simulink model "test"  (R2015a)
settings: Solver=ode3  StartTime=0.0  StopTime=inf  FixedStep=0.01  RelTol=1e-3
undefined symbols (not defined in the file or in its folder): Serial_Port, Standard_Devices
libraries: AAxpcseriallibold x2, xpcseriallib x2, simulink x1, xpcobsoletelib x1, sldrtlib x1
settings Model: SimulationMode=external  Creator=mcshardd  LastModifiedBy=mcshardd
settings SolverCC: EnableConcurrentExecution=on
settings OptimizationCC: BlockReduction=off  OptimizeBlockIOStorage=off  BufferReuse=off  GlobalBufferReuse=off  ExpressionFolding=off  LocalBlockOutputs=off
settings HardwareCC: ProdIntDivRoundTo=Zero  ProdEndianess=LittleEndian  ProdLongLongMode=on  ProdHWDeviceType=Generic->32-bit x86 compatible
settings RTWCC: SystemTargetFile=slrt.tlc  TemplateMakefile=slrt_default_tmf  Description=Simulink Real-Time  RTWCompilerOptimization=on
settings SimulinkRealTimeCC: GeneratePreprocessorConditionals=Disable all

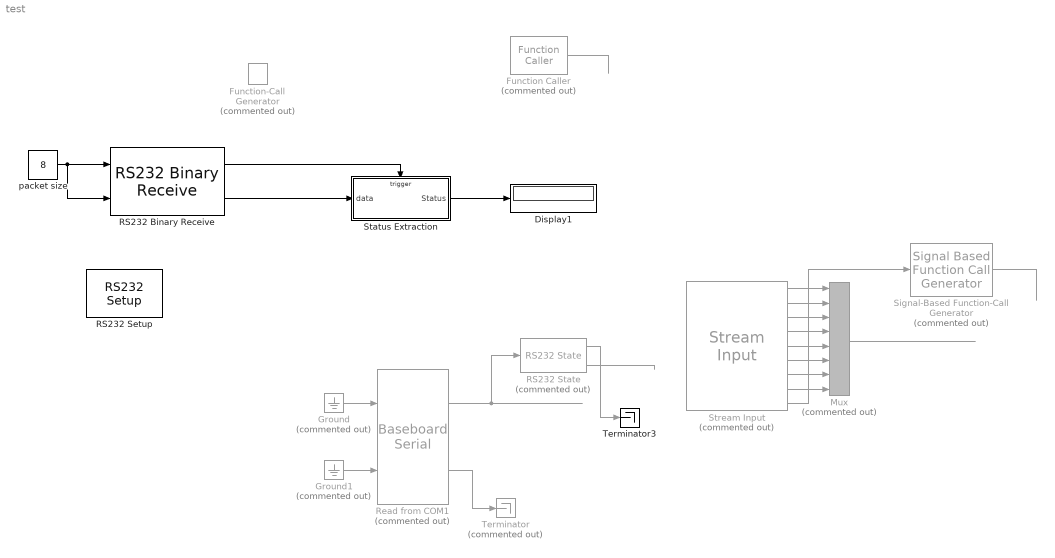
== system test ==
  Display1 : Display
  Function Caller : FunctionCaller  Commented=on  FunctionPrototype=y = f(u)  InputArgumentSpecifications=boolean(1)  OutputArgumentSpecifications=boolean(1)
  Function-Call Generator : simulink/Ports & Subsystems/Function-Call Generator  Commented=on  sample_time=-1  numberOfIterations=1
  Ground : Ground  Commented=on
  Ground1 : Ground  Commented=on
  Mux : Mux  Commented=on  Inputs=8
  RS232 Binary Receive : AAxpcseriallibold/Obsolete/Binary Mode/RS232 Binary Receive  port=COM3  width=8  samptime=-1
  "RS232 Setup " : AAxpcseriallibold/Obsolete/RS232 Setup   port=COM1  baud=19200  dbits=8  sbits=1  parity=None  prot=None  sbuf=2048  rbuf=2048  initstruct=[]  termstruct=[]
  RS232 State : xpcseriallib/RS232 State  Commented=on  overrun=off  parity=off  frame=off  breakint=on
  Read from COM1 : xpcseriallib/Mainboard/Baseboard Serial  Commented=on  group=Receive Setup  port=1  irqnum=4  saddr1=0x3e8  saddr2=0x3e8  config=Custom  baud1=115200  parity1=None  ndata1=8  nstop1=1  fifomode1=16 deep  rlevel1=half full  automode1=off  xmtfifosize1=2048  xmtdatatype1=8 bit uint null terminated  rcvfifosize1=2048  rcvmaxread1=2048  rcvminread1=1  rcvusedelim1=on  rcvdelim1=13  rcvdatatype1=8 bit int null terminated  rcvsampletime1=-1  baud2=115200  parity2=None  ndata2=8  nstop2=1  fifomode2=16 deep  rlevel2=half full  automode2=off  xmtfifosize2=1024  xmtdatatype2=8 bit uint null terminated  rcvfifosize2=1024  rcvmaxread2=1024  rcvminread2=1  rcvusedelim2=on  rcvdelim2=13  rcvdatatype2=count+16 bit uint  rcvsampletime2=.01
      link override FIFO read 1: enable=off
  Signal-Based Function-Call Generator : SignalBasedFunctionCallGenerator  Commented=on  GenerateFunctionCallUpon=Trigger from port tr
      settings: InputPortMap=u1
  Status Extraction : Subsystem  TreatAsAtomicUnit=on
  Stream Input : sldrtlib/Stream Input  Commented=on  SampleTime=0.1  MaxMissedTicks=10  ShowMissedTicks=off  YieldWhenWaiting=off  DrvName=Standard_Devices/Serial_Port  DrvAddress=1  DrvOptions=[115200 8 0 0 0 0 0 0]  DataTypes={'double' 'double' 'double' 'double' 'double' 'double' 'double' 'double'}  FormatString="'%f %f %f %f %f %f  %f %f'"  Terminator={'\r', '\n'}  ShowReady=on  ShowError=off
      settings: AttributesFormatString=Standard Devices\nSerial Port [1h]
  Terminator : Terminator  Commented=on
  Terminator3 : Terminator
  packet size : Constant  Value=8
  wires:
  Status Extraction/1(Status) -> Display1/1
  Stream Input/1 -> Mux/1
  Stream Input/2 -> Mux/2
  Stream Input/3 -> Mux/3
  Stream Input/4 -> Mux/4
  Stream Input/5 -> Mux/5
  Stream Input/6 -> Mux/6
  Stream Input/7 -> Mux/7
  Stream Input/8 -> Mux/8
  Stream Input/9 -> Signal-Based Function-Call Generator/1
  Mux/1 -> ?
  Signal-Based Function-Call Generator/1 -> ?
  Read from COM1/1 -> RS232 State/1
  Ground/1 -> Read from COM1/1
  Read from COM1/2 -> Terminator/1
  Ground1/1 -> Read from COM1/2
  RS232 State/2 -> ?
  RS232 State/1 -> Terminator3/1
  Function Caller/1 -> ?
  packet size/1 -> RS232 Binary Receive/2, RS232 Binary Receive/1
  RS232 Binary Receive/2 -> Status Extraction/1(data)
  RS232 Binary Receive/1 -> Status Extraction/Trigger

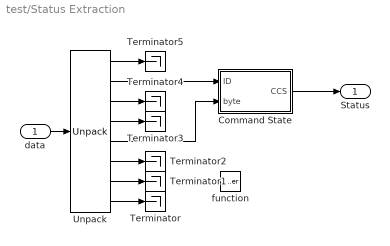
== system test/Status Extraction ==
  data : Inport
  function : TriggerPort  TriggerType=function-call  OutputDataType=int8
  Command State : MATLAB Function  TreatAsAtomicUnit=on
  Terminator{,1..5} (6 alike) : Terminator
  Unpack : xpcobsoletelib/Utilities/Unpack   dimensions={1,1,1,1,1,1,1,1}  datatypes={'uint8','uint8','uint8','uint8','uint8','uint8','uint8','uint8'}  byteAlign=1
  Status : Outport
  wires:
  data/1 -> Unpack/1
  Command State/1(CCS) -> Status/1
  Unpack/5 -> Command State/2(byte)
  Unpack/2 -> Command State/1(ID)
  Unpack/8 -> Terminator/1
  Unpack/1 -> Terminator5/1
  Unpack/3 -> Terminator4/1
  Unpack/4 -> Terminator3/1
  Unpack/6 -> Terminator2/1
  Unpack/7 -> Terminator1/1

== matlab function test/Status Extraction/Command State ==
  data: ID input; CCS output; byte input
function CCS = fcn(ID, byte)
% This block supports an embeddable subset of the MATLAB language.
% See the help menu for details. 
% outputs the command channel state (CCS) given status output

% first check that have proper status message
% ID = 10 for SSC status info
if ID==10
    if byte==2
        out=1;
    elseif byte==4;
        out=2;
    elseif byte==6
        out=3;
    else
        out=0;
    end
else
    out=4;
end
CCS = out;
